simulink model "week1_p2"  (R2020a)
settings: Solver=VariableStepAuto  StartTime=0.0  StopTime=10.0  RelTol=1e-3
undefined symbols (not defined in the file): B, K1, K2, M2
settings Model: Creator=prabhudevmaddipudi  LastModifiedBy=prabhudevmaddipudi

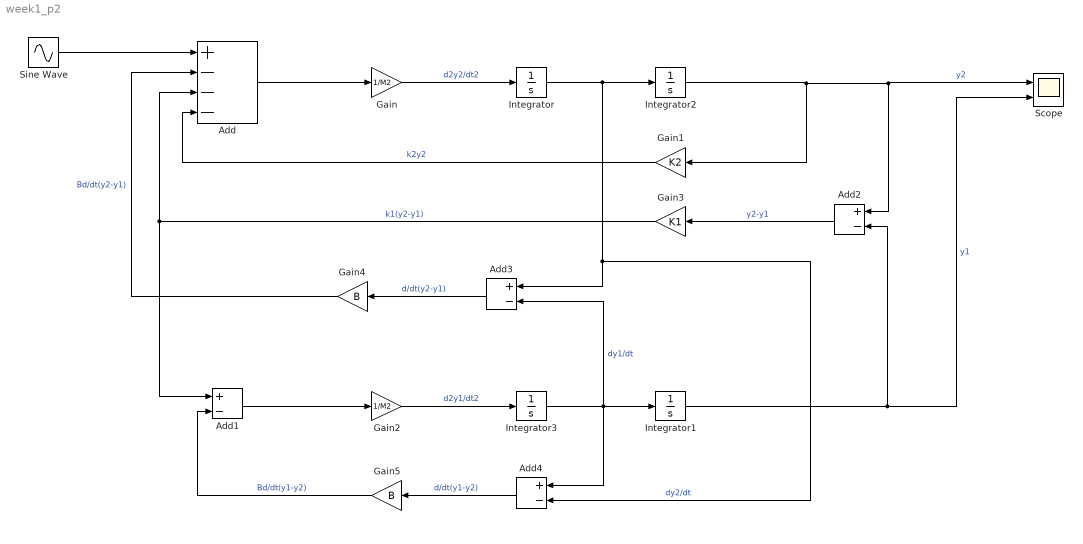
== system week1_p2 ==
  Add : Sum  Inputs=+---
  Add{1..4} (4 alike) : Sum  Inputs=+-
  Gain : Gain  Gain=1/M2
  Gain1 : Gain  Gain=K2
  Gain2 : Gain  Gain=1/M2
  Gain3 : Gain  Gain=K1
  Gain4 : Gain  Gain=B
  Gain5 : Gain  Gain=B
  Integrator{,1..3} (4 alike) : Integrator
  Scope : Scope  NumInputPorts=2
  Sine Wave : Sin  SampleTime=0
  wires:
  Gain1/1 -> Add/4  "k2y2"
  Gain/1 -> Integrator/1  "d2y2/dt2"
  Add3/1 -> Gain4/1  "d/dt(y2-y1)"
  Integrator/1 -> Add4/2, Add3/1, Integrator2/1  "dy2/dt"
  Add2/1 -> Gain3/1  "y2-y1"
  Gain5/1 -> Add1/2  "Bd/dt(y1-y2)"
  Gain3/1 -> Add1/1, Add/3  "k1(y2-y1)"
  Add/1 -> Gain/1
  Sine Wave/1 -> Add/1
  Gain2/1 -> Integrator3/1  "d2y1/dt2"
  Add1/1 -> Gain2/1
  Integrator1/1 -> Scope/2, Add2/2  "y1"
  Integrator3/1 -> Add4/1, Add3/2, Integrator1/1  "dy1/dt"
  Add4/1 -> Gain5/1  "d/dt(y1-y2)"
  Gain4/1 -> Add/2  "Bd/dt(y2-y1)"
  Integrator2/1 -> Add2/1, Scope/1, Gain1/1  "y2"
